simulink model "zad1"  (R2017a)
settings: Solver=VariableStepAuto  StartTime=0.0  StopTime=16.0  RelTol=1e-3
settings Model: Creator=DoktorHax  LastModifiedBy=DoktorHax

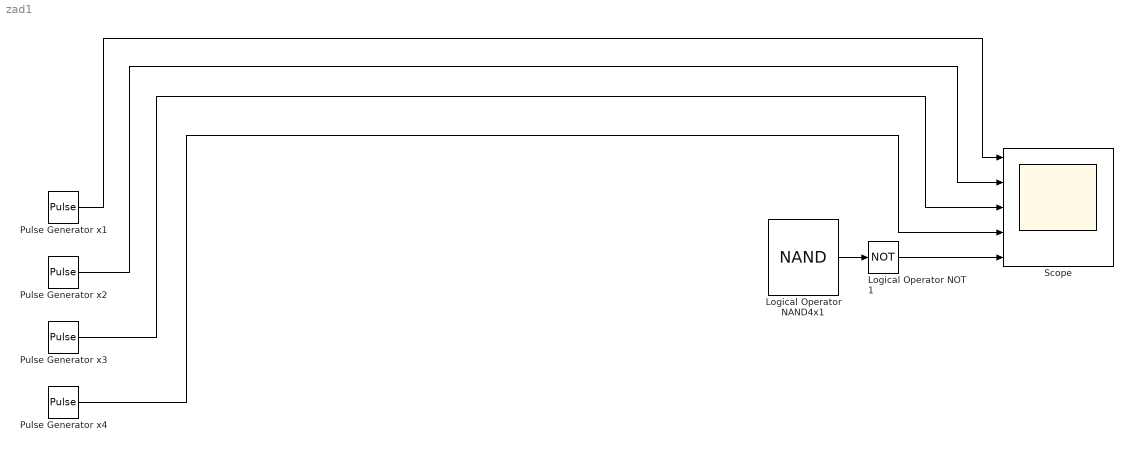
== system zad1 ==
  Logical Operator NAND4x1 : Logic  Operator=NAND  Inputs=4  AllPortsSameDT=off  OutDataTypeStr=boolean
  Logical Operator NOT 1 : Logic  Operator=NOT  AllPortsSameDT=off  OutDataTypeStr=boolean
  Pulse Generator x1 : DiscretePulseGenerator  PulseType=Time based  PulseWidth=50
  Pulse Generator x2 : DiscretePulseGenerator  PulseType=Time based  Period=4  PulseWidth=50
  Pulse Generator x3 : DiscretePulseGenerator  PulseType=Time based  Period=8  PulseWidth=50
  Pulse Generator x4 : DiscretePulseGenerator  PulseType=Time based  Period=16  PulseWidth=50
  Scope : Scope  NumInputPorts=5
  wires:
  Pulse Generator x1/1 -> Scope/1
  Pulse Generator x2/1 -> Scope/2
  Pulse Generator x3/1 -> Scope/3
  Pulse Generator x4/1 -> Scope/4
  Logical Operator NAND4x1/1 -> Logical Operator NOT 1/1
  Logical Operator NOT 1/1 -> Scope/5
